simulink model "test"  (R2018a)
settings: Solver=FixedStepAuto  StartTime=0.0  StopTime=21545  FixedStep=1  MaxStep=4000.0  RelTol=1e-3
settings Model: Creator=Cédric  LastModifiedBy=Cédric

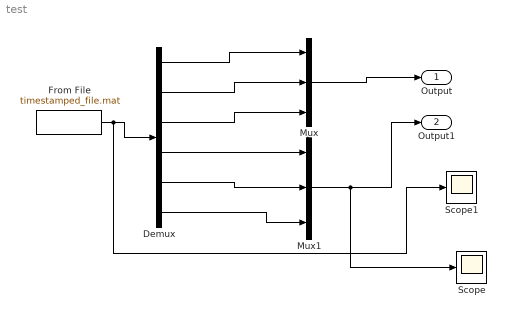
== system test ==
  Demux : Demux  Outputs=6
  From File : FromFile  FileName=timestamped_file.mat  SampleTime=1
  Mux : Mux  Inputs=3
  Mux1 : Mux  Inputs=3
  Scope : Scope
  Scope1 : Scope
  Output : Outport  SignalName=SatVel_J2000
  Output1 : Outport  Port=2  SignalName=SatPos_J2000
  wires:
  Mux/1 -> Output/1
  Mux1/1 -> Scope/1, Output1/1
  From File/1 -> Scope1/1, Demux/1
  Demux/1 -> Mux/1
  Demux/2 -> Mux/2
  Demux/3 -> Mux/3
  Demux/4 -> Mux1/1
  Demux/5 -> Mux1/2
  Demux/6 -> Mux1/3
